simulink model "ardupilotsailboat"  (R2022b)
settings: Solver=VariableStepAuto  StartTime=0.0  StopTime=250  RelTol=1e-3
values from neighbouring files (symbols this model uses):
  Ixx = 1/120 * pi * rho * L * B * T * (4*T^2 + B^2)    (= 0.835683076278)    [parameterCalculations.m]
  m = 2    [parameterCalculations.m]
  m11 = m*k11    [parameterCalculations.m]
  m22 = m*k22    [parameterCalculations.m]
  Yv = Yv * (u^2)/(U^2)    (= -23.3298597446)    [parameterCalculations.m]
undefined symbols (not defined in the file or in its folder): Waypoints
libraries: cstblocks x6, simulink x1, vrlib x1
(part 2 of 2)

== matlab function ardupilotsailboat/MATLAB Function6 ==
  data: r input; u input; Xh output; v input; Yh output; Kh output; Nh output; Frh output; phi input
function [Xh,Yh,Kh,Nh,Frh] = hullForce(r,u,v,phi)
yh = 0;
zh = -0.1;
xh = 0;
B = 0.125;
rho = 1025;
L = 0.95;
Lwl =0.9;
g = 9.81;
delta = 0.5 * 4/3 * B * L * 0.125 * pi;
% from the hull
v_ahu = -u + r*yh;
v_ahv = (-v-r*xh + 0*zh)/cos(0);
v_ah = sqrt(v_ahu^2 + v_ahv^2);
alpha_ah = atan2(real(v_ahv),real(-v_ahu));
%Frh = resistancehull(u);
Re = (abs(v_ahu)*Lwl)/(abs(v_ahv));
Cf = 0.075 / (log(Re)-2)^2;
Frh = 0.5 * rho * u^2 * Cf * (0.5*delta);

Xh = -Frh*cos(alpha_ah)*1;
if abs(Xh)>15
    if Xh >0
        Xh=15;
    else
        Xh = -15;
    end
end
Yh = -Frh*sin(alpha_ah)*cos(phi);

if abs(Yh)>15
    if Yh >0
        Yh=15;
    else
        Yh = -15;
    end
end
Kh = Frh*sin(alpha_ah)*cos(phi)*zh;

if abs(Kh)>15
    if Kh >0
        Kh=15;
    else
        Kh = -15;
    end
end
Nh = -Frh*sin(alpha_ah)*cos(0)*xh;
%D_hull = [Frh*cos(alpha_ah);-Frh*sin(alpha_ah)*cos(phi); Frh*sin(alpha_ah)*cos(phi)*par.zh; -Frh*sin(alpha_ah)*cos(phi)*par.xh];


function F = resistancehull(alpha_a)

xdata = linspace(0,2.6,13); % every 0.5m/s
ydata = [0 6.0018e-04 0.0039*0.0039 0.0127*0.0127 0.0306*0.0306 0.0625*0.0625 0.1157*0.1157 0.2002*0.2002 0.3304*0.3304 0.5274*0.5274 0.8219*0.8 1.2606*0.9 1.9151];

% interpolation
if alpha_a <= 1.3
    F = interp1(xdata,ydata,alpha_a,'pchip');
else
    F = interp1(xdata,ydata,alpha_a,'pchip','extrap');
end

== matlab function ardupilotsailboat/Subsystem8/MATLAB Function19 ==
  data: y output; v input; u input; y1 output
function [y,y1]     = beta(v,u)
% Beta Reference Angle
y=0;
y1 = real(asin(complex(v/sqrt(v^2+u^2))));

== matlab function ardupilotsailboat/MATLAB Function1 ==
  data: y output; psi input; currentState input; nextState output
function [y,nextState]      = zigzagPsi(psi,currentState)

switch currentState
    case 0
        if(psi>(20/180*pi))
            nextState=1;
        else
            nextState=0;
        end
        y=21/180*pi;
    case 1 
        if (psi<-(20/180*pi))
            nextState=0;
        else
            nextState=1;
        end
        y=-21/180*pi;
    otherwise
    y=0;
    nextState=0;
end

== matlab function ardupilotsailboat/Subsystem7/MATLAB Function1 ==
  data: y output; psi input; wind_direction input; alpha_aw output; u input; v input; wind_velocity input; r input; V_aw output
function [y,alpha_aw,V_aw] = sailAngle(psi,wind_direction,u,v,wind_velocity,r)

% CoE of the sail
xs = 0;
ys = 0;
zs = 0.6;
v_t = [ wind_velocity*cos(wind_direction); wind_velocity*sin(wind_direction); 0 ];
R1 = [ cos(-psi) -sin(-psi) 0; sin(-psi) cos(-psi) 0; 0 0 1];
R2 = [ 1 0 0 ; 0 1 0; 0 0 1];
v_tb = R2*R1*v_t; % wind expressed in the body frame
V_in = [ u ; v ; 0 ];
V_awb = v_tb - V_in - cross([0;0;r],[xs;ys;zs]);
V_awu = V_awb(1);
V_awv = V_awb(2);
V_aw = V_awb(1)^2 + V_awb(2)^2;
alpha_aw = atan2(real(V_awv),real(-V_awu));

y=  0.5 * alpha_aw;

== matlab function ardupilotsailboat/MATLAB Function7 ==
  data: y output; r input; currentState input; nextState output
function [y,nextState]      = zigzag(r,currentState)
% Beta Reference Angle

switch currentState
    case 0
        if(r==1)
        nextState=1;
        else 
            nextState=0;
        end
        y=-15/180*pi;
    case 1
        if(r==1)
        nextState=0;
        else 
            nextState=1;
        end
        y=15/180*pi;
    otherwise
        y=-15/180*pi;
        nextState=0;
end

== matlab function ardupilotsailboat/Subsystem1/MATLAB Function1 ==
  data: awa input; psi input; y output
function y = controlAngle(awa,psi)
if psi<-2*pi
    psi=psi+2*pi;
end
if psi>2*pi
    psi=psi-2*pi;
end
if awa<-pi
    awa=awa+pi;
end
if awa>pi
    awa=awa-pi;
end

y = -awa+psi;

== matlab function ardupilotsailboat/MATLAB Function8 ==
  data: y output; psi input; state input
function y      = zigzagPsi(psi,state)
% Beta Reference Angle
if psi<-15 && state == 0
    y=1;
elseif psi>15 && state == 1
    y=1;
else 
    y=0;
end

== matlab function ardupilotsailboat/Subsystem1/MATLAB Function2 ==
  data: x1 input; y1 input; u input; y output; us input; u1 output
function [y,u1] = controlAngle(x1,y1,u,us)
ys=0;
if x1>=0 && y1>=0
    ys=u;
elseif x1>=0 && y1<=0
        ys=pi-u;
elseif x1==0 && y1>0
        ys=-pi;
elseif x1==0 && y1<0
        ys=pi;
elseif y1==0 && x1>0
        ys=pi/2;
elseif y1==0 && x1<0
        ys=-pi/2;
elseif x1<0 && y1>0
    ys=-u-pi;
elseif x1<0 && y1<0
    ys=-pi+u;
else
    ys=u;
end
if (ys-us)<-pi
    %y = ys+2*pi;
elseif (ys-us)>pi
   % y=ys-2*pi;
else
    y=ys;
end
y=ys;
u1=u;

== matlab function ardupilotsailboat/Subsystem1/MATLAB Function13 ==
  data: u input; v input; psi input; psiTrack input; uTrack output; trackDistanceToWaypoint input; closeToWaypoint output
function[uTrack,closeToWaypoint]   = trackVelocity(u,v,psi,psiTrack,trackDistanceToWaypoint)
% Calculate track velocity of sailboat

% Velocity Vector
U = sqrt(u^2+v^2);
psiU = atan(v/u);

psiA = psi + psiU;

uTrack = U * cos(psiTrack + psiA);
closeToWaypoint = 0;
if (trackDistanceToWaypoint/abs(uTrack))<15
    closeToWaypoint = 1;
end

== matlab function ardupilotsailboat/Subsystem1/MATLAB Function10 ==
  data: state input; y output
function y = stopSimulation(state)
if state== 6
    y=1;
else
    y=0;
end

== matlab function ardupilotsailboat/Subsystem1/MATLAB Function14 ==
  data: closeToWaypoint input; theta input; thetaDot input; side output; switchSide output
function[side, switchSide]   = orientSailboat(closeToWaypoint, theta, thetaDot)
% Orientate sailboat so that it passes waypoint with its port side
% Port: 0 
% Starboard: 1 

if closeToWaypoint==1
           if theta > 0 
               if thetaDot > 0 
                   % Port tack and port side of waypoint
                   % Do nothing
                   switchSide = 0;
                   side = 0;
               elseif thetaDot < 0 
                   % Starboard tack but port side of waypoint
                   % Switch tack
                   switchSide=1;
                   side = 1;
               else 
                   switchSide=2;
                   side=2;
               end
           elseif theta < 0
               if thetaDot> 0 
                   % Port tack and starboard side of waypoint
                   % Switch Tack
                   switchSide = 0;
                   side = 0;
               elseif thetaDot < 0 
                        % Starboard tack and starboard side of waypoint
                        % Switch Tack
                        switchSide = 1;
                        side = 1;
               else
                   switchSide=2;
                   side=2;
               end
           else
               switchSide=2;
               side=2;
           end
else
    switchSide=2;
    side=2;
end

== matlab function ardupilotsailboat/Subsystem1/MATLAB Function11 ==
  data: xw input; yw input; xs input; p_w output; ys input; xcw input; ycw input; theta output; pwc input; pwn output; thetaP input
function [p_w,theta,pwn] = passedWaypoint(xw,yw,xs,ys,xcw,ycw,pwc,thetaP)
% Checking is sailboat has passed waypoint while sailing into the wind
switch pwc
    case 0
        if (ys-ycw)~= 0 
            theta = atan(abs(xs-xcw)/abs(ys-ycw));
            pwn=1;
        else 
            pwn=0;
            theta=0;
        end
    case 1
        theta=thetaP;
        pwn=1;
    otherwise
    theta=thetaP;
    pwn=0;
end

p_w=0;
if xw>0 
% Angle between sail
    if (xcw-xs)<0 
        % Waypoint passed in x positive
        p_w=1;
        if(ycw-ys)<0
            % Waypoint passed in both x and y positive direction
            theta = pi + theta;
        else
            % Waypoint passed in positive x and negative y
            theta = -theta;
        end
    end 
else
    if(xcw-xs)>0 
        % Waypoint passed in x negative
        p_w=1;
        if(ycw-ys)>0
           % Waypoint passed in both x and y negative direction
        else
           % Waypoint passed in negative x and positive y
           theta= pi - theta;
        end
   end
end

if p_w==1
    
end

== matlab function ardupilotsailboat/Subsystem1/MATLAB Function12 ==
  data: xs input; ys input; x input; y input; dist input; dist output
function dist   = travelDistance(xs,ys,x,y,dist)
% Distance Sailboat travelled

dist = dist + sqrt((xs-x)^2+(ys-y)^2);

== matlab function ardupilotsailboat/Subsystem1/MATLAB Function18 ==
  data: angle input; nextState output; currentState input
function nextState    = tack_Side(angle,currentState)
% Calculate when to tack back to waypoint

switch currentState
    case 1
        % In zone 1 can go to zone 2 and 4
        if angle < 0
            nextState=4;
        elseif angle > 15
            nextState=2;
        else 
            nextState=1;
        end
    case 2
       % In zone 2 can go to zone 3 and 1
        if angle < 15
            nextState=1;
        elseif angle > 30
            nextState=3;
        else 
            nextState=2;
        end
    case 3
        % In zone 3 can go to zone 2
        if angle < 30
            nextState=2;
        else 
            nextState=3;
        end
    case 4
       % In zone 4 can go to zone 5 and 1
        if angle > 0
            nextState=1;
        elseif angle < -15
            nextState=5;
        else 
            nextState=4;
        end
    case 5
       % In zone 5 can go to zone 6 and 4
        if angle < -30
            nextState=6;
        elseif angle >-15
            nextState=4;
        else
            nextState=5;
        end
    case 6
        % In zone 6 can go to zone 5
        if angle > -30
            nextState=5;
        else 
            nextState=6;
        end
    otherwise
        nextState=1;

end

== matlab function ardupilotsailboat/Subsystem1/MATLAB Function3 ==
  data: pathTrajectory input; y output; tack input; tackDistance output; tackLeft output; tackRight output; WA input; xtrack input; nextTackType output; indirectTackSide input; zone input; currentTackType input; currentState output; noGoAngle input; tackType input; XtrackDistance input; passedWaypoint input; pwTrajectory input; switchSide input; closeToWay input
function [y,tackDistance, tackLeft,tackRight,nextTackType,currentState]  = headingController(pathTrajectory,tack,WA,xtrack,indirectTackSide,zone,currentTackType,noGoAngle,tackType,XtrackDistance,passedWaypoint,pwTrajectory,switchSide,closeToWay)
% Heading State Machine

% Type of Tacks
% Direct = 1
% Indirect = 2
% Zones = 3

tackDistance = XtrackDistance;
if tack==0 && passedWaypoint==0
    currentState = 0;
elseif passedWaypoint==1 && (tackType==1 || tackType==2) 
    currentState = 4;
else
    % Switch between Direct and Indirect Tack and Zone Tack
    currentState = tackType;
    
end
switch currentState
    
    % Normail State 
    case 0
        y = pathTrajectory;
        nextTackType=1;
        tackLeft=0;
        tackRight=0;

    % Direct Tacking State
    case 1
       switch currentTackType
           case 1
               y=WA*180/pi+noGoAngle;
               tackRight=1;
               tackLeft=0;
               if(xtrack>tackDistance)
                   nextTackType=0;
               else
                   nextTackType=1;
               end
               
           case 0 
               y=WA*180/pi-noGoAngle;
               tackRight=0;
               tackLeft=1;
               if (xtrack<-tackDistance)
                   nextTackType=1;
               else 
                   nextTackType=0;
               end
           otherwise
               nextTackType=1;
               y=WA*180/pi+45;
               tackLeft=1;
               tackRight=0;
       end
    
    % Indirect Tacking State
    case 2
        if indirectTackSide==0
             y=WA*180/pi+noGoAngle;
        else
             y=WA*180/pi-noGoAngle;
        end
        nextTackType=1;
        tackLeft=0;
        tackRight=0;

    % Zone Tacking State
    case 3
        switch zone
            case 1
                if currentTackType==0
                    tackLeft=1;
                    tackRight=0;
                    y=WA*180/pi-noGoAngle;
                    nextTackType=0;
                else
                    tackLeft=0;
                    tackRight=1;
                    y=WA*180/pi+noGoAngle;
                    nextTackType=1;
                end

            case 2
                if currentTackType==0
                    tackLeft=1;
                    tackRight=0;
                    y=WA*180/pi-noGoAngle;
                    nextTackType=0;
                else
                    tackLeft=0;
                    tackRight=1;
                    y=WA*180/pi+noGoAngle;
                    nextTackType=1;
                end

            case 3
                % If boat is forced in zone 3 sail past lay lines and only
                % when one has passed the lay lines sail to waypoint
                y = pathTrajectory;
                tackLeft=1;
                nextTackType=0;
                tackRight=0;
            
            case 4
                if currentTackType==0
                    tackLeft=1;
                    tackRight=0;
                    y=WA*180/pi-noGoAngle;
                    nextTackType=0;
                else
                    tackLeft=0;
                    tackRight=1;
                    y=WA*180/pi+noGoAngle;
                    nextTackType=1;
                end

            case 5
                if currentTackType==0
                    tackLeft=1;
                    tackRight=0;
                    y=WA*180/pi-noGoAngle;
                    nextTackType=0;
                else
                    tackLeft=0;
                    tackRight=1;
                    y=WA*180/pi+noGoAngle;
                    nextTackType=1;
                end

            case 6
                % Same as zone 3 just opposite tack
                y = pathTrajectory;
                tackLeft=0;
                nextTackType=1;
                tackRight=1;

            otherwise
                y = pathTrajectory;
                nextTackType=0;
                tackLeft=1;
                tackRight=0;
        end

    case 4
        y = pwTrajectory;
        tackLeft=0;
        nextTackType=1;
        tackRight=1;

    otherwise
        y=0;
        nextTackType=2;
        tackLeft=0;
        tackRight=0;

end
if currentState==3
    if tackLeft==1
         y=WA*180/pi-noGoAngle;
         nextTackType=0;
    else
         y=WA*180/pi+noGoAngle;
         nextTackType=1;
    end
end
if currentState~=0
    if switchSide==1 && closeToWay==1
       nextTackType=1;
    end
end

== matlab function ardupilotsailboat/Subsystem1/MATLAB Function4 ==
  data: R input; nextState output; currentWaypoint output; currentState input
function [nextState,currentWaypoint]  = wayPointController(R,currentState)
% Waypoint switching
% With each added waypoint another case should be added
switch currentState
    % First waypoint
    case 0
        % Check if waypoint lies within radius of acceptance
        if(R==1)
            % Switch current Waypoint to next waypoint
            nextState=1;
            currentWaypoint=1;
        % Waypoint not reached
        else
            nextState=0;
            currentWaypoint=0;
        end
    case 1
        % Check if waypoint lies within radius of acceptance
        if(R==1)
            % Switch current Waypoint to next waypoint
            nextState=2;
            currentWaypoint=2;
       % Waypoint not reached
       else
            nextState=currentState;
            currentWaypoint=1;
       end
    case 2
       % Check if waypoint lies within radius of acceptance
       if(R==1)
            % Switch current Waypoint to next waypoint
            nextState=3;
            currentWaypoint=3;
       % Waypoint not reached
       else
            nextState=currentState;
            currentWaypoint=2;
       end
     case 3
       % Check if waypoint lies within radius of acceptance
       if(R==1)
            % Switch current Waypoint to next waypoint
            nextState=4;
            currentWaypoint=4;
       % Waypoint not reached 
       else
            nextState=currentState;
            currentWaypoint=3;
       end
     case 4
       % Check if waypoint lies within radius of acceptance
       if(R==1)
            % Switch current Waypoint to next waypoint
            nextState=5;
            currentWaypoint=5;
       % Waypoint not reached
       else
            nextState=currentState;
            currentWaypoint=4;
       end
       case 5
       % Check if waypoint lies within radius of acceptance
       if(R==1)
            % Switch current Waypoint to next waypoint
            nextState=6;
            currentWaypoint=6;
       % Waypoint not reached
       else
            nextState=currentState;
            currentWaypoint=5;
       end
       case 6
       % Check if waypoint lies within radius of acceptance
       if(R==1)
            % Switch current Waypoint to next waypoint
            nextState=0;
            currentWaypoint=0;
       % Waypoint not reached
       else
            nextState=currentState;
            currentWaypoint=6;
       end
    otherwise
        nextState=0;
        currentWaypoint=0;
end

== matlab function ardupilotsailboat/Subsystem1/MATLAB Function5 ==
  data: xWaypoint input; yWaypoint input; xBoat input; yBoat input; R input; acceptance output; dist output
function [acceptance,dist]   = circleOfAcceptanceController(xWaypoint,yWaypoint,xBoat,yBoat,R)
dist = sqrt((abs(xWaypoint-xBoat))^2+(abs(yWaypoint-yBoat))^2);
    if (sqrt((abs(xWaypoint-xBoat))^2+(abs(yWaypoint-yBoat))^2)<R)
        acceptance=1;
    else
        acceptance=0;
    end
end

== matlab function ardupilotsailboat/Subsystem1/MATLAB Function6 ==
  data: xw input; yw input; xwp input; y output; ywp input
function y  = distanceToWaypoint(xw,yw,xwp,ywp)
% Calculate distance to waypoint
y = (sqrt((ywp-yw)^2+(xwp-xw)^2))/2;

== matlab function ardupilotsailboat/Subsystem1/MATLAB Function7 ==
  data: wa input; y output; psi input; w output; p output; awa output
function [y,w,p,awa]   = apparentWindAngle(wa,psi)
% Calculate Apparent Wind Angle

if psi> pi
    psi= psi-2*pi;
else
    if psi<-pi
    psi=psi+2*pi;
    end
end
awa = psi-wa;
p=psi;
w= wa;

if abs(awa)<pi/4
    y=1;
else

    y=0;
end

== matlab function ardupilotsailboat/Subsystem1/MATLAB Function8 ==
  data: x1 input; y1 input; u input; y output; us input
function y = controlAngle(x1,y1,u,us)
ys=0;
if x1>=0 && y1>=0
    ys=u;
elseif x1>=0 && y1<=0
        ys=pi-u;
elseif x1==0 && y1>0
        ys=0;
elseif x1==0 && y1<0
        ys=pi;
elseif y1==0 && x1>0
        ys=pi/2;
elseif y1==0 && x1<0
        ys=-pi/2;
elseif x1<0 && y1>0
    ys=-u;
elseif x1<0 && y1<0
    ys=-pi+u;
else
    ys=u;
end
if (ys-us)<-pi
    y = ys+2*pi;
elseif (ys-us)>pi
    y=ys-2*pi;
else
    y=ys;
end

== matlab function ardupilotsailboat/Subsystem1/MATLAB Function9 ==
  data: angle output; dist input; xtrack input; currentState input; tack output; nextState output; windDirection input; wayPointHeading input
function [angle,tack,nextState]  = tackAngle(dist,xtrack,currentState,windDirection,wayPointHeading)
% Calculate when to tack back to waypoint
if dist ~= 0
    angle = atan(xtrack/dist);
else
    angle=0;
end

if windDirection > pi
    windDirection = windDirection - pi;
else
    if windDirection < -pi
        windDirection = windDirection + pi;
    end
end

if wayPointHeading > pi
    wayPointHeading = wayPointHeading - pi;
else
    if wayPointHeading < -pi
        wayPointHeading = wayPointHeading + pi;
    end
end

angle = angle * (180/pi) - (windDirection-wayPointHeading);

% tack == 0 is left tack
% tack == 1 is right tack
switch currentState
    case 0
        tack=0;
        if angle>=45
            nextState=1;
        else
            nextState=0;
        end
    case 1
        tack=1;
        if angle<=-45
            nextState=0;
        else
            nextState=1;
        end

    otherwise
        tack=0;
        nextState=0;

end

== matlab function ardupilotsailboat/Subsystem8/MATLAB Function ==
  data: u input; y output; max input
function y = fcn(u,max)
if u>max
    u=max;
else 
    if u<-max
        u=-max;
    end
end
y = u;

== matlab function ardupilotsailboat/Subsystem7/MATLAB Function ==
  data: u input; y output; max input; min input
function y = fcn(u,max,min)
if u>max
    u=max;
else 
    if u<min
        u=min;
    end
end
y = u;

== matlab function ardupilotsailboat/Subsystem8/MATLAB Function1 ==
  data: u input; y output; max input
function y = fcn(u,max)
if u>max
    u=max;
else 
    if u<-max
        u=-max;
    end
end
y = u;

== matlab function ardupilotsailboat/Subsystem3/MATLAB Function14 ==
  data: beta input; wu output; wv output; wr output; t input
function [wu,wv,wr] = WaveForcesandMoments(beta,t)
% Water density (kg/m^2)
rho = 1025;

% Gravity (m/s^2)
g = 9.81;

% Vessel size (m)
L = 1;
B = 0.125;
T = 0.4;

% Vessels Heading

% Wave Specifications
% amplitude(m)
Ai = 0.4;
% length(m)
lamdai = 2.5;
% encounter frequency (rads)
omegai = 0.4;
% random phase (rads)
phii = -pi;

% Wave Component
waveC = Ai * (2*pi)/lamdai * sin(omegai*t + phii);

% u Component
wu = (10^(-6)) * rho * g * B * L * T * cos(beta) * waveC;

% v Component
wv = (10^(-6)) * rho * g * B * L * T * sin(beta) * waveC;

% r Component
wr = (10^(-6)) * 1/24 * rho * g * B * L * (L^2 - B^2) * sin(2*beta) * waveC^2;

== matlab function ardupilotsailboat/Subsystem3/MATLAB Function15 ==
  data: windDirect input; wi_u output; wi_v output; wi_r output; V_w input; psi input; u input; v input
function [wi_u,wi_v,wi_r] = WindForcesandMoments(windDirect,V_w,psi,u,v)
% Air density (kg/m^2)
rho = 1.225;

% Ship Size
L = 2;
B = 0.125;
T = 0.4;

% centroids above the water line of the frontal and lateral projected areas
H_fw = T - 1.2;
H_lw = T - 1.2;
A_fw = B * H_fw;
A_lw = L * H_lw;


% Symmetrical Ship Coeff
c_x = 0.7;
c_y = 0.825;
c_r = 0.125;

% Wind Velocities in x- and y-coordinates
u_w = V_w * cos(windDirect - psi);
v_w = V_w * sin(windDirect - psi);

% Relative wind velocities
u_rw = u - u_w;
v_rw = v - v_w;

% Relative Wind Velocity and direction
V_rw = sqrt(u_rw^2 + v_rw^2);
gamma_rw = -atan(v_rw/u_rw);

% Wind Coeff
C_x = -c_x * cos(gamma_rw);
C_y = c_y * sin(gamma_rw);
C_r = c_r * sin(2*gamma_rw);

% Wind Forces and Moments
wi_u = 0.5 * rho * V_rw *  C_x * A_fw * 10^(-2);
wi_v = 0.5 * rho * V_rw *  C_y * A_lw * 10^(-2);
wi_r = 0.5 * rho * V_rw *  C_r * A_lw * 10^(-2);
